simulink model "controlador_onoff"  (R2022a)
settings: Solver=VariableStepAuto  StartTime=0.0  StopTime=50  RelTol=1e-3
settings Model: Creator=souza  LastModifiedBy=souza

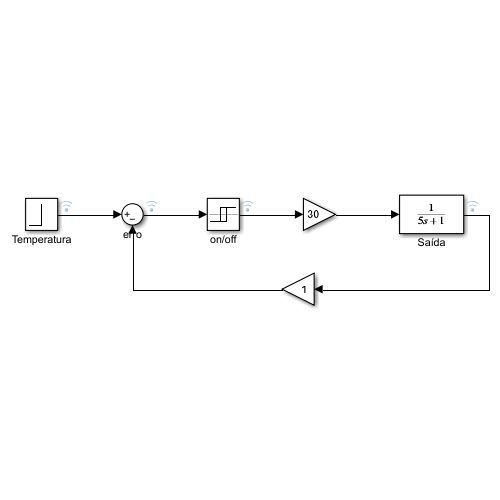
[thumbnail: Simulink's stored preview of the top-level diagram]
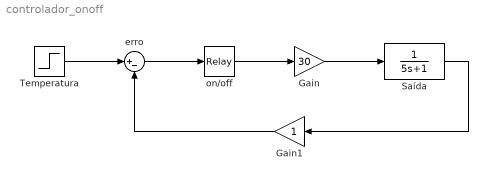
== system controlador_onoff ==
  Gain : Gain  Gain=30
  Gain1 : Gain
  Saída : TransferFcn  Denominator=[5 1]
  Temperatura : Step  Before=20  After=20  SampleTime=0
  erro : Sum  Inputs=|+-
  on/off : Relay  OnSwitchValue=2  OffSwitchValue=-2
  wires:
  Temperatura/1 -> erro/1
  erro/1 -> on/off/1
  on/off/1 -> Gain/1
  Saída/1 -> Gain1/1
  Gain/1 -> Saída/1
  Gain1/1 -> erro/2
